simulink model "FireOrCoastFct"  (R2021a)
settings: configuration reference "CSRef" (kept outside this file)
model workspace (MAT data in the model file):
  DBCoeff = 1
  alph = 1
undefined symbols (not defined in the file): DB
settings Model: ParameterArgumentNames=DBCoeff,alph  OrderedModelArguments=off  Creator=pkhetarp  LastModifiedBy=pkhetarp
settings ConfigSetRef: SourceName=CSRef  SourceLocation=Base Workspace

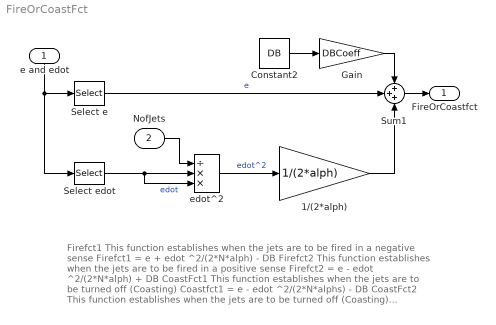
== system FireOrCoastFct ==
  note: Firefct1
      | This function establishes when the jets are to be fired in a negative sense
      | Firefct1 = e + edot ^2/(2*N*alph) - DB
      |
      | Firefct2
      | This function establishes when the jets are to be fired in a positive sense
      | Firefct2 = e - edot ^2/(2*N*alph) + DB
      |
      | CoastFct1
      | This function establishes when the jets are to be turned off (Coasting)
      | Coastfct1 = e - edot ^2/(2*N*alphs) - DB
      |
      | CoastFct2
      | This function establishes when the jets are to be turned off (Coasting)
      | Coastfct2 = e + edot ^2/(2*N*alphs) + DB
  e and edot : Inport  OutDataTypeStr=double  PortDimensions=2  SampleTime=[0.10000000000000001,0]
  NofJets : Inport  Port=2  OutDataTypeStr=double  PortDimensions=1  SampleTime=[0.10000000000000001,0]
  1/(2*alph) : Gain  Gain=1/(2*alph)  SaturateOnIntegerOverflow=on  OutDataTypeStr=Inherit: Same as input  ParamDataTypeStr=Inherit: Same as input
  Constant2 : Constant  Value=DB
  Gain : Gain  Gain=DBCoeff
  Select e : Selector  InputPortWidth=2  IndexOptions=Index vector (dialog)  Indices=[1]  OutputSizes=1
  Select edot : Selector  InputPortWidth=2  IndexOptions=Index vector (dialog)  Indices=[2]  OutputSizes=1
  Sum1 : Sum  Inputs=+++  InputSameDT=on  SaturateOnIntegerOverflow=on  OutDataTypeStr=Inherit: Same as first input
  edot^2 : Product  Inputs=/**  InputSameDT=on  RndMeth=Zero  SaturateOnIntegerOverflow=on  OutDataTypeStr=Inherit: Same as first input
  FireOrCoastfct : Outport  OutDataTypeStr=double  PortDimensions=1  SampleTime=[0.10000000000000001,0]  VectorParamsAs1DForOutWhenUnconnected=off
  wires:
  Sum1/1 -> FireOrCoastfct/1
  Select e/1 -> Sum1/2  "e"
  Constant2/1 -> Gain/1
  1/(2*alph)/1 -> Sum1/3
  e and edot/1 -> Select e/1, Select edot/1
  NofJets/1 -> edot^2/1
  Select edot/1 -> edot^2/2, edot^2/3  "edot"
  edot^2/1 -> 1/(2*alph)/1  "edot^2"
  Gain/1 -> Sum1/1
